simulink subsystem "PvtSubSys_LSM"  (R2020b)
settings: Solver=VariableStepAuto  StartTime=0.0  StopTime=10.0  RelTol=1e-3
values from neighbouring files (symbols this model uses):
  P_LSM_ALC_Enable = 0.0    [LSM_Parameter.sldd]
  P_LSM_DOP_C0_EN_Limit = 0.8    [LSM_Parameter.sldd]
  P_LSM_DOP_C0_out_Limit = 2.0    [LSM_Parameter.sldd]
  P_LSM_DOP_C1_EN_Limit : value not decoded    [LSM_Parameter.sldd]
  P_LSM_DOP_C1_out_Limit : value not decoded    [LSM_Parameter.sldd]
  P_LSM_DOP_C1AndC2_Lim_X : value not decoded    [LSM_Parameter.sldd]
  P_LSM_DOP_C2_EN_Limit : value not decoded    [LSM_Parameter.sldd]
  P_LSM_DOP_C2_out_Limit : value not decoded    [LSM_Parameter.sldd]
  P_LSM_DOP_In_Pre2Dop_Dis = 1.0    [LSM_Parameter.sldd]
  P_LSM_DOP_Out_Pre2Dop_Dis = 2.0    [LSM_Parameter.sldd]
  P_LSM_DOP_PreDis_X : value not decoded    [LSM_Parameter.sldd]
  P_LSM_DOP_PreDis_Y : value not decoded    [LSM_Parameter.sldd]
  P_LSM_DOPValid_CheckTime = 0.06    [LSM_Parameter.sldd]
  P_LSM_DoubleLine_Curr2Cent_Dislimit = 0.5    [LSM_Parameter.sldd]
  P_LSM_DoubleLine_Dop2Cent_Dislimit = 0.5    [LSM_Parameter.sldd]
  P_LSM_DoubleLine_DOPOut_C1 : value not decoded    [LSM_Parameter.sldd]
  P_LSM_DoubleLine_Pre2Cent_Dislimit = 1.0    [LSM_Parameter.sldd]
  P_LSM_IFV2CenterAxis = 0.0    [LSM_Parameter.sldd]
  P_LSM_IFV2RearAxis = 0.0    [LSM_Parameter.sldd]
  P_LSM_LineSTD_Limit = 0.15    [LSM_Parameter.sldd]
  P_LSM_NOH_Switch = 0.0    [LSM_Parameter.sldd]
  P_LSM_Pre_t = 0.0    [LSM_Parameter.sldd]
  P_LSM_SingleLine_Cent2Edge_Dislimit = 100.0    [LSM_Parameter.sldd]
  P_LSM_SingleLine_Curr2Cent_Dislimit = 0.2    [LSM_Parameter.sldd]
  P_LSM_SingleLine_Dop2Cent_Dislimit = 0.2    [LSM_Parameter.sldd]
  P_LSM_SingleLine_DOPOut_C1 : value not decoded    [LSM_Parameter.sldd]
  P_LSM_SingleLine_Pre2Cent_Dislimit = 0.5    [LSM_Parameter.sldd]
undefined symbols (not defined in the file or in its folder): P_LSM_LineWijCal_C12, P_LSM_LineWijCal_C13, P_LSM_PosLineLcFac
libraries: simulink x92, TrueDurationTime x2
(part 7 of 9)

== matlab function PvtSubSys_LSM/Subsystem/TargetLineCalc_20ms/TargetLineCalc/NOA ==
  data: LeftEn input boolean size=1; RightEn input boolean size=1; RFM_LineL1_Valid input uint8 size=1; RFM_LineL1_A0 input single size=1; RFM_LineL1_A1 input single size=1; RFM_LineL1_A2 input single size=1; RFM_LineL1_A3 input single size=1; RFM_LineL1_Range input single size=1; RFM_LineL2_Valid input uint8 size=1; RFM_LineL2_A0 input single size=1; RFM_LineL2_A1 input single size=1; RFM_LineL2_A2 input single size=1; RFM_LineL2_A3 input single size=1; RFM_LineL2_Range input single size=1; RFM_LineR1_Valid input uint8 size=1; RFM_LineR1_A0 input single size=1; RFM_LineR1_A1 input single size=1; RFM_LineR1_A2 input single size=1; RFM_LineR1_A3 input single size=1; RFM_LineR1_Range input single size=1; RFM_LineR2_Valid input uint8 size=1; RFM_LineR2_A0 input single size=1; RFM_LineR2_A1 input single size=1; RFM_LineR2_A2 input single size=1; RFM_LineR2_A3 input single size=1; RFM_LineR2_Range input single size=1; Exit_Valid input uint8 size=1; Exit_A0 input single size=1; Exit_A1 input single size=1; Exit_A2 input single size=1; Exit_A3 input single size=1; Exit_Range input single size=1; Exit_Start input; RFM_LineCL_Valid input uint8 size=1; RFM_LineCL_A0 input single size=1; RFM_LineCL_A1 input single size=1; RFM_LineCL_A2 input single size=1; RFM_LineCL_A3 input single size=1; RFM_LineCL_Range input single size=1; HWASts input uint8 size=1; HWAStsK1 input uint8 size=1; PilotSts input uint8 size=1; LaneChange input uint8 size=1; PilotRoadSts input uint8 size=1; DistanceLim input single size=1; HWALineValid output boolean size=1; MoveIDK1 input int8 size=1; HWALineC3 output single size=1; HWALineC2 output single size=1; HWALineC1 output single size=1; HWALineC0 output single size=1; HWARange output single size=1; HWALeLineValid output boolean size=1; HWALeLineC3 output single size=1; HWALeLineC2 output single size=1; HWALeLineC1 output single size=1; HWALeLineC0 output single size=1; HWALeRange output single size=1; HWARiLineValid output boolean size=1; HWARiLineC3 output single size=1; HWARiLineC2 output single size=1; HWARiLineC1 output single size=1; HWARiLineC0 output single size=1; HWARiRange output single size=1; MoveID output int8 size=1; LockIDK1 input int8 size=1; LockID output int8 size=1; Lock_counterK1 input uint8; Lock_counter output uint8
function [HWALineValid,HWALineC3,HWALineC2,HWALineC1,HWALineC0,HWARange,...
    HWALeLineValid,HWALeLineC3,HWALeLineC2,HWALeLineC1,HWALeLineC0,HWALeRange,...
    HWARiLineValid,HWARiLineC3,HWARiLineC2,HWARiLineC1,HWARiLineC0,HWARiRange,...
    MoveID,LockID,Lock_counter] = fcn(LeftEn,RightEn,RFM_LineL1_Valid,RFM_LineL1_A0,RFM_LineL1_A1,RFM_LineL1_A2,RFM_LineL1_A3,RFM_LineL1_Range,...
    RFM_LineL2_Valid,RFM_LineL2_A0,RFM_LineL2_A1,RFM_LineL2_A2,RFM_LineL2_A3,RFM_LineL2_Range,...
    RFM_LineR1_Valid,RFM_LineR1_A0,RFM_LineR1_A1,RFM_LineR1_A2,RFM_LineR1_A3,RFM_LineR1_Range,...
    RFM_LineR2_Valid,RFM_LineR2_A0,RFM_LineR2_A1,RFM_LineR2_A2,RFM_LineR2_A3,RFM_LineR2_Range,...
    Exit_Valid,Exit_A0,Exit_A1,Exit_A2,Exit_A3,Exit_Range,Exit_Start,...
    RFM_LineCL_Valid,RFM_LineCL_A0,RFM_LineCL_A1,RFM_LineCL_A2,RFM_LineCL_A3,RFM_LineCL_Range,HWASts,HWAStsK1,...
    PilotSts,LaneChange,PilotRoadSts,DistanceLim,MoveIDK1,LockIDK1,Lock_counterK1)
HWALineValid = false;
HWALineC3 = single(0);
HWALineC2 = single(0);
HWALineC1 = single(0);
HWALineC0 = single(0);
HWARange = single(0);

HWALeLineValid = false;
HWALeLineC3 = single(0);
HWALeLineC2 = single(0);
HWALeLineC1 = single(0);
HWALeLineC0 = single(0);
HWALeRange = single(0);

HWARiLineValid = false;
HWARiLineC3 = single(0);
HWARiLineC2 = single(0);
HWARiLineC1 = single(0);
HWARiLineC0 = single(0);
HWARiRange = single(0);

MoveID = MoveIDK1;
LockID = LockIDK1;
Lock_counter = max(Lock_counterK1-uint8(1),uint8(0));
if Lock_counter==0
    LockID = int8(0);
end

if (HWASts==1)||(HWASts==7)||(HWASts==0)||HWASts==2
    MoveID = int8(0);
end
Error=false;

%% NOH
if PilotSts~=0
    if HWASts==1||HWASts==2
        if RFM_LineCL_Valid>0
            HWALineValid = true;
            HWALineC3 = RFM_LineCL_A3;
            HWALineC2 = RFM_LineCL_A2;
            HWALineC1 = RFM_LineCL_A1;
            HWALineC0 = RFM_LineCL_A0;
            HWARange = RFM_LineCL_Range;
        end
        if RFM_LineL1_Valid>0&&RFM_LineL2_Valid>0&&...
                (RFM_LineL1_Range>DistanceLim||RFM_LineL2_Range>DistanceLim)&&LeftEn
            HWALeLineValid = true;
            HWALeLineC3 = 0.5*(RFM_LineL1_A3+RFM_LineL2_A3);
            HWALeLineC2 = 0.5*(RFM_LineL1_A2+RFM_LineL2_A2);
            HWALeLineC1 = 0.5*(RFM_LineL1_A1+RFM_LineL2_A1);
            HWALeLineC0 = 0.5*(RFM_LineL1_A0+RFM_LineL2_A0);
            HWALeRange = 0.5*(RFM_LineL1_Range+RFM_LineL2_Range);
        end
        if RFM_LineR1_Valid>0&&RFM_LineR2_Valid>0&&...
                (RFM_LineR1_Range>DistanceLim||RFM_LineR2_Range>DistanceLim)&&RightEn
            HWARiLineValid = true;
            HWARiLineC3 = 0.5*(RFM_LineR1_A3+RFM_LineR2_A3);
            HWARiLineC2 = 0.5*(RFM_LineR1_A2+RFM_LineR2_A2);
            HWARiLineC1 = 0.5*(RFM_LineR1_A1+RFM_LineR2_A1);
            HWARiLineC0 = 0.5*(RFM_LineR1_A0+RFM_LineR2_A0);
            HWARiRange = 0.5*(RFM_LineR1_Range+RFM_LineR2_Range);
        end
    end
    if PilotRoadSts==8&&Exit_Valid           %汇出（未行驶到汇出线）
        if Exit_Start>30
            HWALineValid = true;
            HWALineC3 = RFM_LineCL_A3;
            HWALineC2 = RFM_LineCL_A2;
            HWALineC1 = RFM_LineCL_A1;
            HWALineC0 = RFM_LineCL_A0;
            HWARange = RFM_LineCL_Range;
        elseif Exit_Start>16
            temp_x = [0.5*Exit_Start,Exit_Start,Exit_Start+single(10),Exit_Start+single(30)];
            y1 = RFM_LineCL_A0+RFM_LineCL_A1*temp_x(1)+RFM_LineCL_A2*temp_x(1)^2+RFM_LineCL_A3*temp_x(1)^3;
            y3 = Exit_A0+Exit_A1*temp_x(3)+Exit_A2*temp_x(3)^2+Exit_A3*temp_x(3)^3;
            if y3>0
                y2 = min(1,0.4*y3);
            else
                y2 = max(-1,0.4*y3);
            end
            y4 = Exit_A0+Exit_A1*temp_x(4)+Exit_A2*temp_x(4)^2+Exit_A3*temp_x(4)^3;
            temp_y = [y1,y2,y3,y4];
            [HWALineC3,HWALineC2,HWALineC1,HWALineC0] = pl(temp_x,temp_y);
            HWALineValid = true;
            HWARange = Exit_Start+single(40);
        else
            HWALineValid = true;
            HWALineC3 = Exit_A3;
            HWALineC2 = Exit_A2;
            HWALineC1 = Exit_A1;
            HWALineC0 = Exit_A0;
            HWARange = Exit_Range;
        end
    elseif PilotRoadSts==19&&Exit_Valid         % 汇出（行驶到汇出线）
        HWALineValid = true;
        HWALineC3 = Exit_A3;
        HWALineC2 = Exit_A2;
        HWALineC1 = Exit_A1;
        HWALineC0 = Exit_A0;
        HWARange = Exit_Range;
    elseif HWASts==3 || HWASts==11 || HWASts==12       %巡航
        MoveID = int8(0);
        if HWAStsK1==5 || HWAStsK1==6
            Lock_counter = uint8(250);
            LockID = int8(0);
        end
        if Lock_counter>0
            if LaneChange==1
                LockID = LockID + int8(1);
            end
            if LaneChange==2
                LockID = LockID - int8(1);
            end
        else
            LockID = int8(0);
        end
        if LockID==1
            if RFM_LineR1_Valid>0&&RFM_LineR2_Valid>0&&...
                    (RFM_LineR1_Range>DistanceLim||RFM_LineR2_Range>DistanceLim)
                HWALineValid = true;
                HWALineC3 = 0.5*(RFM_LineR1_A3+RFM_LineR2_A3);
                HWALineC2 = 0.5*(RFM_LineR1_A2+RFM_LineR2_A2);
                HWALineC1 = 0.5*(RFM_LineR1_A1+RFM_LineR2_A1);
                HWALineC0 = 0.5*(RFM_LineR1_A0+RFM_LineR2_A0);
                HWARange = 0.5*(RFM_LineR1_Range+RFM_LineR2_Range);
            elseif RFM_LineR1_Valid>0&&...
                    RFM_LineR1_Range>DistanceLim
                HWALineValid = true;
                HWALineC3 = RFM_LineR1_A3;
                HWALineC2 = RFM_LineR1_A2;
                HWALineC1 = RFM_LineR1_A1;
                HWALineC0 = RFM_LineR1_A0 - 1.875*sqrt(single(1) + RFM_LineR1_A1*RFM_LineR1_A1);
                HWARange = RFM_LineR1_Range;
            elseif RFM_LineR2_Valid>0&&...
                    RFM_LineR2_Range>DistanceLim
                HWALineValid = true;
                HWALineC3 = RFM_LineR2_A3;
                HWALineC2 = RFM_LineR2_A2;
                HWALineC1 = RFM_LineR2_A1;
                HWALineC0 = RFM_LineR2_A0 + 1.875*sqrt(single(1) + RFM_LineR2_A1*RFM_LineR2_A1);
                HWARange = RFM_LineR2_Range;
            end
        elseif LockID==-1
            if RFM_LineL1_Valid>0&&RFM_LineL2_Valid>0&&...
                    (RFM_LineL1_Range>DistanceLim||RFM_LineL2_Range>DistanceLim)
                HWALineValid = true;
                HWALineC3 = 0.5*(RFM_LineL1_A3+RFM_LineL2_A3);
                HWALineC2 = 0.5*(RFM_LineL1_A2+RFM_LineL2_A2);
                HWALineC1 = 0.5*(RFM_LineL1_A1+RFM_LineL2_A1);
                HWALineC0 = 0.5*(RFM_LineL1_A0+RFM_LineL2_A0);
                HWARange = 0.5*(RFM_LineL1_Range+RFM_LineL2_Range);
            elseif RFM_LineL1_Valid>0&&...
                    RFM_LineL1_Range>DistanceLim
                HWALineValid = true;
                HWALineC3 = RFM_LineL1_A3;
                HWALineC2 = RFM_LineL1_A2;
                HWALineC1 = RFM_LineL1_A1;
                HWALineC0 = RFM_LineL1_A0 - 1.875*sqrt(single(1) + RFM_LineL1_A1*RFM_LineL1_A1);
                HWARange = RFM_LineL1_Range;
            elseif RFM_LineL2_Valid>0&&...
                    RFM_LineL2_Range>DistanceLim
                HWALineValid = true;
                HWALineC3 = RFM_LineL2_A3;
                HWALineC2 = RFM_LineL2_A2;
                HWALineC1 = RFM_LineL2_A1;
                HWALineC0 = RFM_LineL2_A0 + 1.875*sqrt(single(1) + RFM_LineL2_A1*RFM_LineL2_A1);
                HWARange = RFM_LineL2_Range;
            end
        elseif LockID==0
            HWALineValid = true;
            HWALineC3 = RFM_LineCL_A3;
            HWALineC2 = RFM_LineCL_A2;
            HWALineC1 = RFM_LineCL_A1;
            HWALineC0 = RFM_LineCL_A0;
            HWARange = RFM_LineCL_Range;
        end
    elseif HWASts == 5                     %左换道
        if HWAStsK1~=5
            MoveID = MoveID - int8(1);
        end
        if LaneChange==1
            MoveID = MoveID + int8(1);
        end
        if LaneChange==2
            MoveID = MoveID - int8(1);
        end
        if (MoveID>=1)||(MoveID<=-2)
            Error = true;
        end
        if Error==false
            if MoveID==-1
                if RFM_LineL1_Valid>0&&RFM_LineL2_Valid>0&&...
                        (RFM_LineL1_Range>DistanceLim||RFM_LineL2_Range>DistanceLim)
                    HWALineValid = true;
                    HWALineC3 = 0.5*(RFM_LineL1_A3+RFM_LineL2_A3);
                    HWALineC2 = 0.5*(RFM_LineL1_A2+RFM_LineL2_A2);
                    HWALineC1 = 0.5*(RFM_LineL1_A1+RFM_LineL2_A1);
                    HWALineC0 = 0.5*(RFM_LineL1_A0+RFM_LineL2_A0);
                    HWARange = 0.5*(RFM_LineL1_Range+RFM_LineL2_Range);
                    
                    HWALeLineValid = true;
                    HWALeLineC3 = 0.5*(RFM_LineL1_A3+RFM_LineL2_A3);
                    HWALeLineC2 = 0.5*(RFM_LineL1_A2+RFM_LineL2_A2);
                    HWALeLineC1 = 0.5*(RFM_LineL1_A1+RFM_LineL2_A1);
                    HWALeLineC0 = 0.5*(RFM_LineL1_A0+RFM_LineL2_A0);
                    HWALeRange = 0.5*(RFM_LineL1_Range+RFM_LineL2_Range);
                elseif RFM_LineL1_Valid>0&&...
                        RFM_LineL1_Range>DistanceLim
                    HWALineValid = true;
                    HWALineC3 = RFM_LineL1_A3;
                    HWALineC2 = RFM_LineL1_A2;
                    HWALineC1 = RFM_LineL1_A1;
                    HWALineC0 = RFM_LineL1_A0 - 1.875*sqrt(single(1) + RFM_LineL1_A1*RFM_LineL1_A1);
                    HWARange = RFM_LineL1_Range;
                    
                    HWALeLineValid = true;
                    HWALeLineC3 = RFM_LineL1_A3;
                    HWALeLineC2 = RFM_LineL1_A2;
                    HWALeLineC1 = RFM_LineL1_A1;
                    HWALeLineC0 = RFM_LineL1_A0 - 1.875*sqrt(single(1) + RFM_LineL1_A1*RFM_LineL1_A1);
                    HWALeRange = RFM_LineL1_Range;
                elseif RFM_LineL2_Valid>0&&...
                        RFM_LineL2_Range>DistanceLim
                    HWALineValid = true;
                    HWALineC3 = RFM_LineL2_A3;
                    HWALineC2 = RFM_LineL2_A2;
                    HWALineC1 = RFM_LineL2_A1;
                    HWALineC0 = RFM_LineL2_A0 + 1.875*sqrt(single(1) + RFM_LineL2_A1*RFM_LineL2_A1);
                    HWARange = RFM_LineL2_Range;
                    HWALeLineValid = true;
                    HWALeLineC3 = RFM_LineL2_A3;
                    HWALeLineC2 = RFM_LineL2_A2;
                    HWALeLineC1 = RFM_LineL2_A1;
                    HWALeLineC0 = RFM_LineL2_A0 + 1.875*sqrt(single(1) + RFM_LineL2_A1*RFM_LineL2_A1);
                    HWALeRange = RFM_LineL2_Range;
                end
                HWARiLineValid = true;
                HWARiLineC3 = RFM_LineCL_A3;
                HWARiLineC2 = RFM_LineCL_A2;
                HWARiLineC1 = RFM_LineCL_A1;
                HWARiLineC0 = RFM_LineCL_A0;
                HWARiRange = RFM_LineCL_Range;
            elseif MoveID==0
                HWALineValid = true;
                HWALineC3 = RFM_LineCL_A3;
                HWALineC2 = RFM_LineCL_A2;
                HWALineC1 = RFM_LineCL_A1;
                HWALineC0 = RFM_LineCL_A0;
                HWARange = RFM_LineCL_Range;
            end
        end
    elseif HWASts==6                                     %右换道
        if HWAStsK1~=6
            MoveID = MoveID + int8(1);
        end
        if LaneChange==1
            MoveID = MoveID + int8(1);
        end
        if LaneChange==2
            MoveID = MoveID - int8(1);
        end
        if (MoveID>=2)||(MoveID<=-1)
            Error = true;
        end
        if Error==false
            if MoveID==1
                if RFM_LineR1_Valid>0&&RFM_LineR2_Valid>0&&...
                        (RFM_LineR1_Range>DistanceLim||RFM_LineR2_Range>DistanceLim)
                    HWALineValid = true;
                    HWALineC3 = 0.5*(RFM_LineR1_A3+RFM_LineR2_A3);
                    HWALineC2 = 0.5*(RFM_LineR1_A2+RFM_LineR2_A2);
                    HWALineC1 = 0.5*(RFM_LineR1_A1+RFM_LineR2_A1);
                    HWALineC0 = 0.5*(RFM_LineR1_A0+RFM_LineR2_A0);
                    HWARange = 0.5*(RFM_LineR1_Range+RFM_LineR2_Range);
                    
                    HWARiLineValid = true;
                    HWARiLineC3 = 0.5*(RFM_LineR1_A3+RFM_LineR2_A3);
                    HWARiLineC2 = 0.5*(RFM_LineR1_A2+RFM_LineR2_A2);
                    HWARiLineC1 = 0.5*(RFM_LineR1_A1+RFM_LineR2_A1);
                    HWARiLineC0 = 0.5*(RFM_LineR1_A0+RFM_LineR2_A0);
                    HWARiRange = 0.5*(RFM_LineR1_Range+RFM_LineR2_Range);
                elseif RFM_LineR1_Valid>0&&...
                        RFM_LineR1_Range>DistanceLim
                    HWALineValid = true;
                    HWALineC3 = RFM_LineR1_A3;
                    HWALineC2 = RFM_LineR1_A2;
                    HWALineC1 = RFM_LineR1_A1;
                    HWALineC0 = RFM_LineR1_A0 - 1.875*sqrt(single(1) + RFM_LineR1_A1*RFM_LineR1_A1);
                    HWARange = RFM_LineR1_Range;
                    
                    HWARiLineValid = true;
                    HWARiLineC3 = RFM_LineR1_A3;
                    HWARiLineC2 = RFM_LineR1_A2;
                    HWARiLineC1 = RFM_LineR1_A1;
                    HWARiLineC0 = RFM_LineR1_A0 - 1.875*sqrt(single(1) + RFM_LineR1_A1*RFM_LineR1_A1);
                    HWARiRange = RFM_LineR1_Range;
                elseif RFM_LineR2_Valid>0&&...
                        RFM_LineR2_Range>DistanceLim
                    HWALineValid = true;
                    HWALineC3 = RFM_LineR2_A3;
                    HWALineC2 = RFM_LineR2_A2;
                    HWALineC1 = RFM_LineR2_A1;
                    HWALineC0 = RFM_LineR2_A0 + 1.875*sqrt(single(1) + RFM_LineR2_A1*RFM_LineR2_A1);
                    HWARange = RFM_LineR2_Range;
                    HWARiLineValid = true;
                    HWARiLineC3 = RFM_LineR2_A3;
                    HWARiLineC2 = RFM_LineR2_A2;
                    HWARiLineC1 = RFM_LineR2_A1;
                    HWARiLineC0 = RFM_LineR2_A0 + 1.875*sqrt(single(1) + RFM_LineR2_A1*RFM_LineR2_A1);
                    HWARiRange = RFM_LineR2_Range;
                end
                HWALeLineValid = true;
                HWALeLineC3 = RFM_LineCL_A3;
                HWALeLineC2 = RFM_LineCL_A2;
                HWALeLineC1 = RFM_LineCL_A1;
                HWALeLineC0 = RFM_LineCL_A0;
                HWALeRange = RFM_LineCL_Range;
            elseif MoveID==0
                HWALineValid = true;
                HWALineC3 = RFM_LineCL_A3;
                HWALineC2 = RFM_LineCL_A2;
                HWALineC1 = RFM_LineCL_A1;
                HWALineC0 = RFM_LineCL_A0;
                HWARange = RFM_LineCL_Range;
            end
        end
    end
end

== matlab function PvtSubSys_LSM/Subsystem/TargetLineCalc_20ms/TargetLineCalc/RoadWidthCalc1 ==
  data: YBranch_b input boolean size=1; VisLineConf input uint8 size=4; a1 input single size=4; a0 input single size=4; LineUpdate input boolean size=1; RoadWidth output single size=1; RoadWidthK1 input single size=1; tLostK1 input single size=1; tLost output single size=1
function [RoadWidth,tLost] = VisRoadWidth(YBranch_b,VisLineConf,a1,a0,LineUpdate,RoadWidthK1,tLostK1)

RoadWidth = RoadWidthK1;
tLost = tLostK1;
Update = false;
temp = single(0);

if LineUpdate
    if (VisLineConf(2)>0)&&(VisLineConf(3)>0)&&(YBranch_b==false)
        if abs(57.3*(atan(a1(2)) - atan(a1(3))))<3
            temp = (a0(2) - a0(3))/sqrt(a1(2)^2 + single(1));
            if (temp>2.5)&&(temp<4.2)
                Update = true;
            end
        end
    end
    if Update
        RoadWidth = 0.1*(temp - RoadWidthK1) + RoadWidthK1;
        tLost = single(0);
    else
        tLost = min(10,tLostK1 + single(0.05));
    end
end

== stateflow chart PvtSubSys_LSM/Subsystem/TargetLineCalc_20ms/TargetLineCalc/Subsystem3/Subsystem/Chart ==
  state init
    PilotRoadSts=PilotRoadSts_init;
  state init1
    PilotRoadSts=19;
  (default) -> init
  init -> init1 : [PilotRoadSts_init==19]
  init1 -> init : [bIsLineExist<2||rExitStub3==1||lExitStub3==1]
  data: PilotRoadSts_init input uint8 size=1; bIsLineExist input uint8 size=1; PilotRoadSts output uint8 size=1; lExitStub3 input boolean size=1; rExitStub3 input boolean size=1

== stateflow chart PvtSubSys_LSM/Subsystem/TargetLineCalc_20ms/TargetLineCalc/Subsystem3/Subsystem/Chart1 ==
  state on
    state CruiseValid2
      PilotRoadSts=18;
      LSM_PilotSPL=uint8(60);
      PilotSPLDist=uint16(0);
      state init
        state Name
          PilotTurnSwSts =0;
        state init4
          PilotTurnSwSts =6;
        state init5
          PilotTurnSwSts =3;
        state init3
          PilotTurnSwSts =7;
        (default) -> on.CruiseValid2.init.Name
        on.CruiseValid2.init.Name -> on.CruiseValid2.init.init3 [order 3] : [FrbRight>0]
        on.CruiseValid2.init.init3 -> on.CruiseValid2.init.Name : [FrbRight==0]
        on.CruiseValid2.init.Name -> on.CruiseValid2.init.init4 [order 1] : [FrbLeft>0]
        on.CruiseValid2.init.init4 -> on.CruiseValid2.init.Name : [FrbLeft==0]
        on.CruiseValid2.init.Name -> on.CruiseValid2.init.init5 [order 2] : [OneLane>0]
        on.CruiseValid2.init.init5 -> on.CruiseValid2.init.Name : [OneLane==0]
      state Name2
        PilotTurnSwSts=1;
      state init1
        PilotTurnSwSts =1;
      state init2
        PilotTurnSwSts =2;
      (default) -> on.CruiseValid2.init
      on.CruiseValid2.init -> on.CruiseValid2.Name2 [order 1] : [Vanish_turnleft>0]
      on.CruiseValid2.Name2 -> on.CruiseValid2.init : [Vanish_turnleft==0]
      on.CruiseValid2.init -> on.CruiseValid2.init1 [order 2] : [CruiseTurn>0&&...
          | TurnLeft>0]
      on.CruiseValid2.init1 -> on.CruiseValid2.init [order 1] : [CruiseTurn==0]
      on.CruiseValid2.init -> on.CruiseValid2.init2 [order 3] : [CruiseTurn>0&&...
          | TurnRight>0]
      on.CruiseValid2.init2 -> on.CruiseValid2.init [order 1] : [CruiseTurn==0]
      on.CruiseValid2.init2 -> on.CruiseValid2.init1 [order 2] : [TurnLeft>0]
      on.CruiseValid2.init1 -> on.CruiseValid2.init2 [order 2] : [TurnRight>0]
    state CruiseValid1
      PilotRoadSts=24;
      LSM_PilotSPL=0xff;
      PilotSPLDist=0xffff;
      state init
        state Name
          PilotTurnSwSts =0;
        state init4
          PilotTurnSwSts =6;
        state init5
          PilotTurnSwSts =3;
        state init3
          PilotTurnSwSts =7;
        (default) -> on.CruiseValid1.init.Name
        on.CruiseValid1.init.Name -> on.CruiseValid1.init.init3 [order 3] : [FrbRight>0]
        on.CruiseValid1.init.init3 -> on.CruiseValid1.init.Name : [FrbRight==0]
        on.CruiseValid1.init.Name -> on.CruiseValid1.init.init4 [order 1] : [FrbLeft>0]
        on.CruiseValid1.init.init4 -> on.CruiseValid1.init.Name : [FrbLeft==0]
        on.CruiseValid1.init.Name -> on.CruiseValid1.init.init5 [order 2] : [OneLane>0]
        on.CruiseValid1.init.init5 -> on.CruiseValid1.init.Name : [OneLane==0]
      state Name2
        PilotTurnSwSts=1;
      state init1
        PilotTurnSwSts =1;
      state init2
        PilotTurnSwSts =2;
      (default) -> on.CruiseValid1.init
      on.CruiseValid1.init -> on.CruiseValid1.Name2 [order 1] : [Vanish_turnleft>0]
      on.CruiseValid1.Name2 -> on.CruiseValid1.init : [Vanish_turnleft==0]
      on.CruiseValid1.init -> on.CruiseValid1.init1 [order 3] : [CruiseTurn>0&&...
          | TurnLeft>0]
      on.CruiseValid1.init1 -> on.CruiseValid1.init [order 1] : [CruiseTurn==0]
      on.CruiseValid1.init -> on.CruiseValid1.init2 [order 2] : [CruiseTurn>0&&...
          | TurnRight>0]
      on.CruiseValid1.init2 -> on.CruiseValid1.init [order 1] : [CruiseTurn==0]
      on.CruiseValid1.init2 -> on.CruiseValid1.init1 [order 2] : [TurnLeft>0]
      on.CruiseValid1.init1 -> on.CruiseValid1.init2 [order 2] : [TurnRight>0]
    state CruiseValid
      PilotRoadSts=17;
      LSM_PilotSPL=0xff;
      PilotSPLDist=0xffff;
      state init
        state Name
          PilotTurnSwSts =0;
        state init4
          PilotTurnSwSts =6;
        state init5
          PilotTurnSwSts =3;
        state init3
          PilotTurnSwSts =7;
        (default) -> on.CruiseValid.init.Name
        on.CruiseValid.init.Name -> on.CruiseValid.init.init3 [order 3] : [FrbRight>0]
        on.CruiseValid.init.init3 -> on.CruiseValid.init.Name : [FrbRight==0]
        on.CruiseValid.init.Name -> on.CruiseValid.init.init4 [order 1] : [FrbLeft>0]
        on.CruiseValid.init.init4 -> on.CruiseValid.init.Name : [FrbLeft==0]
        on.CruiseValid.init.Name -> on.CruiseValid.init.init5 [order 2] : [OneLane>0]
        on.CruiseValid.init.init5 -> on.CruiseValid.init.Name : [OneLane==0]
      state Name2
        PilotTurnSwSts=1;
      state init1
        PilotTurnSwSts =1;
      state init2
        PilotTurnSwSts =2;
      on.CruiseValid.init -> on.CruiseValid.Name2 [order 2] : [Vanish_turnleft>0]
      (default) -> on.CruiseValid.init
      on.CruiseValid.Name2 -> on.CruiseValid.init : [Vanish_turnleft==0]
      on.CruiseValid.init -> on.CruiseValid.init1 [order 1] : [CruiseTurn>0&&...
          | TurnLeft>0]
      on.CruiseValid.init1 -> on.CruiseValid.init [order 1] : [CruiseTurn==0]
      on.CruiseValid.init -> on.CruiseValid.init2 [order 3] : [CruiseTurn>0&&...
          | TurnRight>0]
      on.CruiseValid.init2 -> on.CruiseValid.init [order 1] : [CruiseTurn==0]
      on.CruiseValid.init2 -> on.CruiseValid.init1 [order 2] : [TurnLeft>0]
      on.CruiseValid.init1 -> on.CruiseValid.init2 [order 2] : [TurnRight>0]
    state EntryStub1
      PilotRoadSts=26;
      state Name
        PilotTurnSwSts =1;
      state Name1
        PilotTurnSwSts =4;
      (default) -> on.EntryStub1.Name
      on.EntryStub1.Name -> Name1 : [EntryStub5_TurnLeft==0]
      Name1 -> on.EntryStub1.Name : [EntryStub5_TurnLeft>0]
    state EntryStub2
      PilotTurnSwSts =0;
      PilotRoadSts=25;
    state StubValid
      state EntryStub3
        PilotTurnSwSts =4;
        PilotRoadSts=2;
      state EntryStub4
        PilotTurnSwSts =4;
        PilotRoadSts=1;
      state init
        PilotTurnSwSts =0;
        PilotRoadSts=0;
        LSM_PilotSPL=uint8(60);
        PilotSPLDist=uint16(f_distance);
      state EntryStub1
        PilotTurnSwSts =4;
        PilotRoadSts=2;
      state EntryStub2
        PilotTurnSwSts =4;
        PilotRoadSts=1;
      state Name
        PilotTurnSwSts =2;
        PilotRoadSts=7;
        LSM_PilotSPL=uint8(60);
        PilotSPLDist=uint16(f_distance);
      state LeftStub
        PilotTurnSwSts =1;
        PilotRoadSts=9;
        LSM_PilotSPL=uint8(60);
        PilotSPLDist=uint16(f_distance);
      state Name2
        PilotTurnSwSts =3;
        PilotRoadSts=7;
        LSM_PilotSPL=uint8(60);
        PilotSPLDist=uint16(f_distance);
      state Name3
        PilotTurnSwSts =5;
        PilotRoadSts=8;
        LSM_PilotSPL=uint8(60);
        PilotSPLDist=uint16(f_distance);
      state Name4
        PilotTurnSwSts =2;
        PilotRoadSts=20;
        LSM_PilotSPL=uint8(60);
        PilotSPLDist=uint16(f_distance);
      state CruiseLeft
        PilotTurnSwSts =3;
        PilotRoadSts=9;
        LSM_PilotSPL=uint8(60);
        PilotSPLDist=uint16(f_distance);
      state lExitStub3
        PilotTurnSwSts =1;
        PilotRoadSts=20;
        LSM_PilotSPL=uint8(60);
        PilotSPLDist=uint16(f_distance);
      state lExitStub1
        PilotTurnSwSts =5;
        PilotRoadSts=10;
        LSM_PilotSPL=uint8(60);
        PilotSPLDist=uint16(f_distance);
      state Name5
        PilotTurnSwSts =5;
        PilotRoadSts=19;
        LSM_PilotSPL=uint8(60);
        PilotSPLDist=uint16(f_distance);
      state lExitStub2
        PilotTurnSwSts =5;
        PilotRoadSts=19;
        LSM_PilotSPL=uint8(60);
        PilotSPLDist=uint16(f_distance);
      EntryStub4 -> EntryStub3 [order 1] : [EntryStub3>0]
      (default) -> on.StubValid.init
      EntryStub3 -> EntryStub4 [order 1] : [EntryStub4>0]
      on.StubValid.init -> EntryStub3 [order 2] : [EntryStub3>0]
      EntryStub3 -> on.StubValid.init [order 2] : [EntryStub3==0&&EntryStub4==0]
      on.StubValid.init -> EntryStub4 [order 4] : [EntryStub4>0]
      EntryStub4 -> on.StubValid.init [order 2] : [EntryStub3==0&&EntryStub4==0]
      on.StubValid.init -> on.StubValid.EntryStub1 [order 7] : [EntryStub1>0]
      on.StubValid.EntryStub1 -> on.StubValid.init [order 2] : [EntryStub1==0&&EntryStub2==0]
      on.StubValid.EntryStub1 -> on.StubValid.EntryStub2 [order 1] : [EntryStub2>0]
      on.StubValid.EntryStub2 -> on.StubValid.EntryStub1 [order 1] : [EntryStub1>0]
      on.StubValid.init -> on.StubValid.EntryStub2 [order 8] : [EntryStub2>0]
      on.StubValid.EntryStub2 -> on.StubValid.init [order 2] : [EntryStub1==0&&EntryStub2==0]
      (junction 434) -> on.StubValid.init
      (junction 453) -> on.StubValid.init
      on.StubValid.init -> CruiseLeft [order 5] : [CruiseLeft>0]
      CruiseLeft -> on.StubValid.init [order 3] : [CruiseLeft==0&&...
          | LeftStub==0&&...
          | rExitStub1==0]
      on.StubValid.init -> LeftStub [order 6] : [LeftStub>0]
      LeftStub -> on.StubValid.init [order 2] : [LeftStub==0&&CruiseLeft==0]
      on.StubValid.init -> lExitStub1 [order 10] : [lExitStub1>0]
      lExitStub3 -> on.StubValid.init [order 3] : [lExitStub2==0&&...
          | lExitStub3==0&&...
          | lExitStub1==0]
      (junction 266) -> on.StubValid.init
      (junction 280) -> on.StubValid.init
      on.StubValid.init -> on.StubValid.Name2 [order 3] : [CruiseRight>0]
      on.StubValid.Name2 -> on.StubValid.init [order 3] : [CruiseRight==0&&...
          | RightStub==0&&...
          | rExitStub1==0]
      on.StubValid.init -> on.StubValid.Name [order 1] : [RightStub>0]
      on.StubValid.Name -> on.StubValid.init [order 2] : [RightStub==0&&CruiseRight==0]
      on.StubValid.init -> Name3 [order 9] : [rExitStub1>0]
      Name4 -> on.StubValid.init [order 3] : [rExitStub2==0&&...
          | rExitStub3==0&&...
          | rExitStub1==0]
      on.StubValid.Name -> on.StubValid.Name2 [order 1] : [CruiseRight>0]
      LeftStub -> CruiseLeft [order 1] : [CruiseLeft>0]
      on.StubValid.Name2 -> on.StubValid.Name [order 2] : [RightStub>0]
      CruiseLeft -> LeftStub [order 2] : [LeftStub>0]
      on.StubValid.Name2 -> Name3 [order 1] : [rExitStub1>0]
      Name3 -> Name4 [order 1] : [rExitStub3>0]
      Name3 -> on.StubValid.Name2 [order 3] : [CruiseRight>0]
      CruiseLeft -> lExitStub1 [order 1] : [lExitStub1>0]
      lExitStub1 -> lExitStub3 [order 1] : [lExitStub3>0]
      lExitStub1 -> CruiseLeft [order 3] : [CruiseLeft>0]
      Name4 -> Name3 [order 2] : [rExitStub1>0]
      Name3 -> (junction 280) [order 4] : [CruiseRight==0&&...
          | rExitStub1==0&&...
          | rExitStub3==0&&...
          | rExitStub2==0]
      Name3 -> Name5 [order 2] : [rExitStub2>0]
      Name5 -> Name3 [order 2] : [rExitStub1>0]
      Name5 -> Name4 [order 1] : [rExitStub3>0]
      Name4 -> Name5 [order 1] : [rExitStub2>0]
      lExitStub3 -> lExitStub1 [order 2] : [lExitStub1>0]
      lExitStub1 -> (junction 453) [order 4] : [CruiseLeft==0&&...
          | lExitStub1==0&&...
          | lExitStub3==0&&...
          | lExitStub2==0]
      lExitStub3 -> lExitStub2 [order 1] : [lExitStub2>0]
      lExitStub2 -> lExitStub3 [order 1] : [lExitStub3>0]
      lExitStub1 -> lExitStub2 [order 2] : [lExitStub2>0]
      lExitStub2 -> lExitStub1 [order 2] : [lExitStub1>0]
      Name5 -> (junction 266) [order 3] : [rExitStub2==0&&rExitStub3==0&&rExitStub1==0]
      lExitStub2 -> (junction 434) [order 3] : [lExitStub2==0&&lExitStub3==0&&lExitStub1==0]
    (junction 533) -> (junction 532)
    CruiseValid -> (junction 533) [order 3] : [RoadType~=1&&RoadType~=2]
    (junction 532) -> CruiseValid2
    (junction 527) -> (junction 528)
    (junction 528) -> CruiseValid
    CruiseValid2 -> (junction 527) [order 1] : [RoadType==1]
    on.EntryStub1 -> CruiseValid [order 1] : [CruiseValid>0&&RoadType==1&&EntryStub5==0&&EntryStub6==0]
    CruiseValid -> on.EntryStub1 [order 4] : [EntryStub5>0]
    CruiseValid1 -> CruiseValid2 [order 3] : [RoadType~=1&&RoadType~=2]
    CruiseValid -> CruiseValid1 [order 2] : [RoadType==2]
    on.EntryStub2 -> on.EntryStub1 [order 2] : [EntryStub5>0]
    on.EntryStub1 -> on.EntryStub2 [order 2] : [EntryStub6>0]
    CruiseValid2 -> CruiseValid1 [order 3] : [RoadType==2]
    CruiseValid1 -> CruiseValid [order 2] : [RoadType==1]
    StubValid -> on.EntryStub1 [order 2] : [EntryStub5>0]
    on.EntryStub1 -> StubValid [order 3] : [EntryStub5==0&&EntryStub6==0]
    CruiseValid -> on.EntryStub2 [order 5] : [EntryStub6>0]
    on.EntryStub2 -> CruiseValid [order 1] : [CruiseValid>0&&...
        | RoadType==1&&...
        | EntryStub5==0&&...
        | EntryStub6==0]
    CruiseValid2 -> StubValid [order 2] : [StubValid>0]
    StubValid -> CruiseValid2 [order 5] : [CruiseValid>0&&RoadType~=1&&RoadType~=2&&EntryStub5==0&&EntryStub6==0]
    CruiseValid -> StubValid [order 1] : [StubValid>0]
    StubValid -> CruiseValid [order 1] : [CruiseValid>0&&RoadType==1&&EntryStub5==0&&EntryStub6==0]
    CruiseValid1 -> StubValid [order 1] : [StubValid>0]
    StubValid -> CruiseValid1 [order 4] : [CruiseValid>0&&RoadType==2&&EntryStub5==0&&EntryStub6==0]
    StubValid -> on.EntryStub2 [order 3] : [EntryStub6>0]
    on.EntryStub2 -> StubValid [order 3] : [EntryStub5==0&&EntryStub6==0]
    (default) -> StubValid
  state off1
    PilotTurnSwSts =0;
    PilotRoadSts =0;
    LSM_PilotSPL=0xff;
    PilotSPLDist=0xffff;
  (default) -> off1
  off1 -> on : [i_mapvalid==3&&i_on_nav_path>0]
  on -> off1 : [i_mapvalid~=3||i_on_nav_path==0]
  data: StubValid input boolean size=1; RightStub input boolean size=1; RoadType input uint8 size=1; PilotRoadSts output uint8 size=1; PilotTurnSwSts output uint8 size=1; LeftStub input boolean size=1; CruiseValid input boolean size=1; TurnLeft input boolean size=1; TurnRight input boolean size=1; Vanish_turnleft input boolean size=1; EntryStub1 input boolean size=1; rExitStub1 input boolean size=1; rExitStub2 input boolean size=1; i_mapvalid input uint8 size=1; i_on_nav_path input uint8 size=1; CruiseLeft input boolean size=1; CruiseRight input boolean size=1; f_distance input single size=1; LSM_PilotSPL output uint8 size=1; PilotSPLDist output uint16 size=1; CruiseTurn input boolean size=1; EntryStub2 input boolean size=1; lExitStub1 input boolean size=1; lExitStub2 input boolean size=1; lExitStub3 input boolean size=1; rExitStub3 input boolean size=1; FrbLeft input boolean size=1; FrbRight input boolean size=1; OneLane input boolean size=1; EntryStub3 input; EntryStub4 input; EntryStub5 input; EntryStub6 input; EntryStub5_TurnLeft input

== matlab function PvtSubSys_LSM/Subsystem/TargetLineCalc_20ms/TargetLineCalc/Subsystem3/Subsystem/MATLAB Function ==
  data: NOH_Valid input boolean size=1; PilotSts output uint8 size=1; RoadType input uint8 size=1; rExitStub4_takeover input; lExitStub4_takeover input; EntryStub5_takeover input; Vanish_turnleft_takeover input
function PilotSts = fcn(NOH_Valid,RoadType,rExitStub4_takeover,lExitStub4_takeover,EntryStub5_takeover,Vanish_turnleft_takeover)
PilotSts=uint8(0);
if NOH_Valid == 1
    if RoadType == 1
        PilotSts = uint8(1); %NOH-HW Mode
    end
    if RoadType == 2
        PilotSts = uint8(4); %NOH-City Mode
    end
    if RoadType ~=1 && RoadType ~=2
        PilotSts = uint8(2); %NOH-Ramp Mode
    end
    if rExitStub4_takeover>0 || lExitStub4_takeover>0 || EntryStub5_takeover>0 || Vanish_turnleft_takeover>0
        PilotSts = uint8(3); %NOH-TakeOver
    end
end

== matlab function PvtSubSys_LSM/Subsystem/TargetLineCalc_20ms/TargetLineCalc/Subsystem3/Subsystem2/MATLAB Function ==
  data: nLaneID input uint8 size=1; i_rec_lanes input uint8 size=8; Forbid_TurnRight output boolean size=1; Forbid_TurnLeft output boolean size=1; OneLane output boolean size=1; i_rec_lanes_num input
function [Forbid_TurnRight,Forbid_TurnLeft,OneLane] = fcn(nLaneID,i_rec_lanes,i_rec_lanes_num)

Forbid_TurnRight = false;
Forbid_TurnLeft = false;
OneLane = false;
m=uint8(1);
if i_rec_lanes_num == 1
    if nLaneID==i_rec_lanes(1)
        OneLane = true;
    end
end
if i_rec_lanes_num > 1 
    if i_rec_lanes(1)>1 && nLaneID==i_rec_lanes(1)
        Forbid_TurnLeft = true;
    end

    for i=uint8(1):length(i_rec_lanes)
        if i_rec_lanes(i)>0
            m=i;
        end
    end

    if nLaneID == i_rec_lanes(m)
        Forbid_TurnRight = true;
    end
end

== matlab function PvtSubSys_LSM/Subsystem/TargetLineCalc_20ms/TargetLineCalc/Subsystem3/Subsystem2/Subsystem/MATLAB Function14 ==
  data: u input; y output; i_k input; i output uint8
function [y,i] = fcn(u,i_k)
y = uint8(0);
i = i_k;
if u>2 || u<-2
    i = i+1;
else
    i = uint8(0);
end
if i>10
    y = uint8(1);
end

== matlab function PvtSubSys_LSM/Subsystem/TargetLineCalc_20ms/TargetLineCalc/Subsystem3/Subsystem2/Subsystem1/MATLAB Function14 ==
  data: u input; y output; i_k input; i output uint8
function [y,i] = fcn(u,i_k)
y = uint8(0);
i = i_k;
if u>2 || u<-2
    i = i+1;
else
    i = uint8(0);
end
if i>10
    y = uint8(1);
end

== matlab function PvtSubSys_LSM/Subsystem/TargetLineCalc_20ms/TargetLineCalc/Subsystem3/Subsystem2/Subsystem10/MATLAB Function14 ==
  data: u input; y output; i_k input; i output uint8
function [y,i] = fcn(u,i_k)
y = uint8(0);
i = i_k;
if u>2 || u<-2
    i = i+1;
else
    i = uint8(0);
end
if i>10
    y = uint8(1);
end

== matlab function PvtSubSys_LSM/Subsystem/TargetLineCalc_20ms/TargetLineCalc/Subsystem3/Subsystem2/Subsystem11/MATLAB Function14 ==
  data: u input; y output; i_k input; i output uint8
function [y,i] = fcn(u,i_k)
y = uint8(0);
i = i_k;
if u>2 || u<-2
    i = i+1;
else
    i = uint8(0);
end
if i>10
    y = uint8(1);
end

== matlab function PvtSubSys_LSM/Subsystem/TargetLineCalc_20ms/TargetLineCalc/Subsystem3/Subsystem2/Subsystem12/MATLAB Function14 ==
  data: u input; y output; i_k input; i output uint8
function [y,i] = fcn(u,i_k)
y = uint8(0);
i = i_k;
if u>2 || u<-2
    i = i+1;
else
    i = uint8(0);
end
if i>10
    y = uint8(1);
end

== matlab function PvtSubSys_LSM/Subsystem/TargetLineCalc_20ms/TargetLineCalc/Subsystem3/Subsystem2/Subsystem13/MATLAB Function14 ==
  data: u input; y output; i_k input; i output uint8
function [y,i] = fcn(u,i_k)
y = uint8(0);
i = i_k;
if u>2 || u<-2
    i = i+1;
else
    i = uint8(0);
end
if i>10
    y = uint8(1);
end

== matlab function PvtSubSys_LSM/Subsystem/TargetLineCalc_20ms/TargetLineCalc/Subsystem3/Subsystem2/Subsystem14/MATLAB Function14 ==
  data: u input; y output; i_k input; i output uint8
function [y,i] = fcn(u,i_k)
y = uint8(0);
i = i_k;
if u>2 || u<-2
    i = i+1;
else
    i = uint8(0);
end
if i>10
    y = uint8(1);
end

== matlab function PvtSubSys_LSM/Subsystem/TargetLineCalc_20ms/TargetLineCalc/Subsystem3/Subsystem2/Subsystem15/MATLAB Function14 ==
  data: u input; y output; i_k input; i output uint8
function [y,i] = fcn(u,i_k)
y = uint8(0);
i = i_k;
if u>2 || u<-2
    i = i+1;
else
    i = uint8(0);
end
if i>10
    y = uint8(1);
end

== matlab function PvtSubSys_LSM/Subsystem/TargetLineCalc_20ms/TargetLineCalc/Subsystem3/Subsystem2/Subsystem16/MATLAB Function14 ==
  data: u input; y output; i_k input; i output uint8
function [y,i] = fcn(u,i_k)
y = uint8(0);
i = i_k;
if u>2 || u<-2
    i = i+1;
else
    i = uint8(0);
end
if i>10
    y = uint8(1);
end

== matlab function PvtSubSys_LSM/Subsystem/TargetLineCalc_20ms/TargetLineCalc/Subsystem3/Subsystem2/Subsystem2/MATLAB Function14 ==
  data: u input; y output; i_k input; i output uint8
function [y,i] = fcn(u,i_k)
y = uint8(0);
i = i_k;
if u>2 || u<-2
    i = i+1;
else
    i = uint8(0);
end
if i>10
    y = uint8(1);
end

== matlab function PvtSubSys_LSM/Subsystem/TargetLineCalc_20ms/TargetLineCalc/Subsystem3/Subsystem2/Subsystem3/MATLAB Function14 ==
  data: u input; y output; i_k input; i output uint8
function [y,i] = fcn(u,i_k)
y = uint8(0);
i = i_k;
if u>2 || u<-2
    i = i+1;
else
    i = uint8(0);
end
if i>10
    y = uint8(1);
end

== matlab function PvtSubSys_LSM/Subsystem/TargetLineCalc_20ms/TargetLineCalc/Subsystem3/Subsystem2/Subsystem4/MATLAB Function14 ==
  data: u input; y output; i_k input; i output uint8
function [y,i] = fcn(u,i_k)
y = uint8(0);
i = i_k;
if u>2 || u<-2
    i = i+1;
else
    i = uint8(0);
end
if i>10
    y = uint8(1);
end

== matlab function PvtSubSys_LSM/Subsystem/TargetLineCalc_20ms/TargetLineCalc/Subsystem3/Subsystem2/Subsystem5/MATLAB Function14 ==
  data: u input; y output; i_k input; i output uint8
function [y,i] = fcn(u,i_k)
y = uint8(0);
i = i_k;
if u>2 || u<-2
    i = i+1;
else
    i = uint8(0);
end
if i>10
    y = uint8(1);
end

== matlab function PvtSubSys_LSM/Subsystem/TargetLineCalc_20ms/TargetLineCalc/Subsystem3/Subsystem2/Subsystem6/MATLAB Function14 ==
  data: u input; y output; i_k input; i output uint8
function [y,i] = fcn(u,i_k)
y = uint8(0);
i = i_k;
if u>2 || u<-2
    i = i+1;
else
    i = uint8(0);
end
if i>10
    y = uint8(1);
end

== matlab function PvtSubSys_LSM/Subsystem/TargetLineCalc_20ms/TargetLineCalc/Subsystem3/Subsystem2/Subsystem7/MATLAB Function14 ==
  data: u input; y output; i_k input; i output uint8
function [y,i] = fcn(u,i_k)
y = uint8(0);
i = i_k;
if u>2 || u<-2
    i = i+1;
else
    i = uint8(0);
end
if i>10
    y = uint8(1);
end

== matlab function PvtSubSys_LSM/Subsystem/TargetLineCalc_20ms/TargetLineCalc/Subsystem3/Subsystem2/Subsystem8/MATLAB Function14 ==
  data: u input; y output; i_k input; i output uint8
function [y,i] = fcn(u,i_k)
y = uint8(0);
i = i_k;
if u>2 || u<-2
    i = i+1;
else
    i = uint8(0);
end
if i>10
    y = uint8(1);
end

== matlab function PvtSubSys_LSM/Subsystem/TargetLineCalc_20ms/TargetLineCalc/Subsystem3/Subsystem2/Subsystem9/MATLAB Function14 ==
  data: u input; y output; i_k input; i output uint8
function [y,i] = fcn(u,i_k)
y = uint8(0);
i = i_k;
if u>2 || u<-2
    i = i+1;
else
    i = uint8(0);
end
if i>10
    y = uint8(1);
end

== matlab function PvtSubSys_LSM/Subsystem/TargetLineCalc_20ms/TargetLineCalc/TJA2NOA ==
  data: TJALineValid input boolean size=1; HWALineValid output boolean size=1; TJALineA3 input single size=1; TJALineA2 input single size=1; TJALineA1 input single size=1; TJALineA0 input single size=1; TJALineRange input single size=1; HWALineC3 output single size=1; HWALineC2 output single size=1; HWALineC1 output single size=1; HWALineC0 output single size=1; HWARange output single size=1
function [HWALineValid,HWALineC3,HWALineC2,HWALineC1,HWALineC0,HWARange] =...
    fcn(TJALineValid,TJALineA3,TJALineA2,...
    TJALineA1,TJALineA0,TJALineRange)
HWALineValid = TJALineValid;
HWALineC3 = TJALineA3;
HWALineC2 = TJALineA2;
HWALineC1 = TJALineA1;
HWALineC0 = TJALineA0;
HWARange = TJALineRange;

== matlab function PvtSubSys_LSM/Subsystem/TargetLineCalc_20ms/TargetLineCalc/VisLineFilter5 ==
  data: LeftOffset_b input boolean size=1; RightOffset_b input boolean; LckLock_b input boolean size=1; LckLock_bK1 input boolean size=1; CentLineValid input boolean size=1; CentLineC3 input single size=1; CentLineC2 input single; CentLineC1 input single; CentLineC0 input single; CentLineRange input single; CentLineReliable input single; LeftLineValid input boolean; LeftLineC3 input single; LeftLineC2 input single; LeftLineC1 input single; LeftLineC0 input single; LeftLineRange input single; LeftLineReliable input single; LeftLaneAvail input boolean; RightLineValid input boolean; RightLineC3 input single; RightLineC2 input single; RightLineC1 input single; RightLineC0 input single; RightLineRange input single; RightLineReliable input single; PathValid output boolean; PathA3 output single; PathA2 output single; PathA1 output single; PathA0 output single; PathRange output single; PathReliable output single; RightLaneAvail input boolean; PathLaneAvail output boolean size=3; LockIDK1 input int8; LockID output int8
function [PathValid,PathA3,PathA2,PathA1,PathA0,PathRange,PathReliable,PathLaneAvail,LockID] = ...
    VisFilter(LeftOffset_b,RightOffset_b,LckLock_b,LckLock_bK1,...
    CentLineValid,CentLineC3,CentLineC2,CentLineC1,CentLineC0,CentLineRange,CentLineReliable,...
    LeftLineValid,LeftLineC3,LeftLineC2,LeftLineC1,LeftLineC0,LeftLineRange,LeftLineReliable,LeftLaneAvail,...
    RightLineValid,RightLineC3,RightLineC2,RightLineC1,RightLineC0,RightLineRange,RightLineReliable,RightLaneAvail,LockIDK1)

PathValid = false(3,1);
PathA3 = single(zeros(3,1));
PathA2 = single(zeros(3,1));
PathA1 = single(zeros(3,1));
PathA0 = single(zeros(3,1));
PathRange = single(zeros(3,1));
PathReliable = single(zeros(3,1));
PathLaneAvail = false(3,1);

if LckLock_b
    LockID = LockIDK1;
else
    LockID = int8(0);
end

if (LckLock_b==true)&&(LckLock_bK1==true)
    if LeftOffset_b
        LockID = LockID + int8(1);
    end
    if RightOffset_b
        LockID = LockID + int8(-1);
    end
end

if LockID==int8(1)
    PathValid(2) = RightLineValid;
    PathA3(2) = RightLineC3;
    PathA2(2) = RightLineC2;
    PathA1(2) = RightLineC1;
    PathA0(2) = RightLineC0;
    PathRange(2) = RightLineRange;
    PathReliable(2) = RightLineReliable;
    PathLaneAvail(2) = true;
elseif LockID==int8(-1)
    PathValid(2) = LeftLineValid;
    PathA3(2) = LeftLineC3;
    PathA2(2) = LeftLineC2;
    PathA1(2) = LeftLineC1;
    PathA0(2) = LeftLineC0;
    PathRange(2) = LeftLineRange;
    PathReliable(2) = LeftLineReliable;
    PathLaneAvail(2) = true;
elseif LockID==int8(0)
    PathValid(1) = LeftLineValid;
    PathA3(1) = LeftLineC3;
    PathA2(1) = LeftLineC2;
    PathA1(1) = LeftLineC1;
    PathA0(1) = LeftLineC0;
    PathRange(1) = LeftLineRange;
    PathReliable(1) = LeftLineReliable;
    PathLaneAvail(1) = LeftLaneAvail;
    
    PathValid(2) = CentLineValid;
    PathA3(2) = CentLineC3;
    PathA2(2) = CentLineC2;
    PathA1(2) = CentLineC1;
    PathA0(2) = CentLineC0;
    PathRange(2) = CentLineRange;
    PathReliable(2) = CentLineReliable;
    PathLaneAvail(2) = true;
    
    PathValid(3) = RightLineValid;
    PathA3(3) = RightLineC3;
    PathA2(3) = RightLineC2;
    PathA1(3) = RightLineC1;
    PathA0(3) = RightLineC0;
    PathRange(3) = RightLineRange;
    PathReliable(3) = RightLineReliable;
    PathLaneAvail(3) = RightLaneAvail;
end

== matlab function PvtSubSys_LSM/Subsystem/TargetLineCalc_20ms/TargetLineCalc/TypeConf/MATLAB Function ==
  data: update input; LeftType output uint8 size=1; LeftType_en input uint8 size=1; LeftDLMType_en input uint8 size=1; LeftDECELType_en input uint8; RightType_en input uint8 size=1; RightDLMType_en input uint8 size=1; RightDECELType_en input uint8; LeftColor_en input uint8; LLeftType_en input uint8; LeftTypeK1 input uint8 size=1; LeftDLMTypeK1 input uint8 size=1; LeftDECELTypeK1 input uint8; RightTypeK1 input uint8 size=1; RightDLMTypeK1 input uint8 size=1; LeftDLMType output uint8 size=1; LeftDECELType output; RightType output uint8 size=1; RightDLMType output uint8 size=1; RightDECELTypeK1 input uint8; RightDECELType output; LeftColor_enK1 input uint8; LLeftType_enK1 input uint8; LeftColor output; LLeftType output
function [LeftType,LeftDLMType,LeftDECELType,RightType,RightDLMType,RightDECELType,LeftColor,LLeftType] = ...
    fcn(update,LeftType_en,LeftDLMType_en,LeftDECELType_en,RightType_en,RightDLMType_en,RightDECELType_en,LeftColor_en,LLeftType_en,...
        LeftTypeK1,LeftDLMTypeK1,LeftDECELTypeK1,RightTypeK1,RightDLMTypeK1,RightDECELTypeK1,LeftColor_enK1,LLeftType_enK1)
if update
    LeftType = LeftType_en;
    LeftDLMType = LeftDLMType_en;
    LeftDECELType = LeftDECELType_en;
    RightType = RightType_en;
    RightDLMType = RightDLMType_en;
    RightDECELType = RightDECELType_en;
    LeftColor = LeftColor_en;
    LLeftType = LLeftType_en;
else
    LeftType = LeftTypeK1;
    LeftDLMType = LeftDLMTypeK1;
    LeftDECELType = LeftDECELTypeK1;
    RightType = RightTypeK1;
    RightDLMType = RightDLMTypeK1;
    RightDECELType = RightDECELTypeK1;
    LeftColor = LeftColor_enK1;
    LLeftType = LLeftType_enK1;
end

== matlab function PvtSubSys_LSM/Subsystem/TargetLineCalc_20ms/TargetLineCalc/TypeConf/RoadWidthCalc1 ==
  data: LeftType input uint8 size=1; LeftDLMType input; LeftDECELType input; RightType input uint8 size=1; RightDLMType input; RightDECELType input; Cnt1K1 input uint8 size=1; Cnt2K1 input uint8 size=1; LeftEn output boolean size=1; RightEn output boolean size=1; Cnt1 output uint8 size=1; Cnt2 output uint8 size=1
function [LeftEn,RightEn,Cnt1,Cnt2] = Delay(LeftType,LeftDLMType,LeftDECELType,RightType,RightDLMType,RightDECELType,Cnt1K1,Cnt2K1)
Cnt1 = max(Cnt1K1 - uint8(1),uint8(0));
Cnt2 = max(Cnt2K1 - uint8(1),uint8(0));
if LeftType==1||LeftType==6||(LeftType==3&&(LeftDLMType~=2||LeftDLMType~=4))||(LeftType==5&&(LeftDECELType~=2))
   Cnt1 = uint8(10); 
end
if RightType==1||RightType==6||(RightType==3&&(RightDLMType~=2||RightDLMType~=4))||(RightType==5&&(RightDECELType~=2))
   Cnt2 = uint8(10); 
end

if Cnt1>0
    LeftEn = false;
else
    LeftEn = true;
end

if Cnt2>0
    RightEn = false;
else
    RightEn = true;
end
end

== matlab function PvtSubSys_LSM/Subsystem/TargetLineCalc_20ms/TargetLineCalc/TypeConf1/RoadWidthCalc1 ==
  data: LeftType input uint8 size=1; RightType input uint8 size=1; Cnt1K1 input uint8 size=1; Cnt2K1 input uint8 size=1; LeftEn output boolean size=1; RightEn output boolean size=1; Cnt1 output uint8 size=1; Cnt2 output uint8 size=1
function [LeftEn,RightEn,Cnt1,Cnt2] = Delay(LeftType,RightType,Cnt1K1,Cnt2K1)
Cnt1 = max(Cnt1K1 - uint8(1),uint8(0));
Cnt2 = max(Cnt2K1 - uint8(1),uint8(0));
if LeftType~=2 || LeftType~=4 || LeftType~=6
   Cnt1 = uint8(10); 
end
if RightType~=2 || RightType~=4 || RightType~=6
   Cnt2 = uint8(10); 
end

if Cnt1>0
    LeftEn = false;
else
    LeftEn = true;
end

if Cnt2>0
    RightEn = false;
else
    RightEn = true;
end
end
